simulink model "Furuta_Pendulum_Classical_Controller"  (R2018a)
settings: Solver=VariableStepAuto  StartTime=0.0  StopTime=10.0  RelTol=1e-3
values from neighbouring files (symbols this model uses):
  Ac = [0 1 0 0 ... (first row only)    [BasicModelParameters.m]    (also in ControllerDesign_REV0.m; FurutaPendulum.m = [0 1 0 0; 0 0 -a23 0; 0 0 0 1; 0 0 a43 0]; InvertedPendulumStepResponse.m)
  Bc = transpose([0 b21 0 -b41])    [BasicModelParameters.m]    (also in ControllerDesign_REV0.m; FurutaPendulum.m = [0; b21; 0; -b41]; InvertedPendulumStepResponse.m)
  Cc = [1 0 0 0 ... (first row only)    [BasicModelParameters.m]    (also in ControllerDesign_REV0.m; FurutaPendulum.m = [1 0 0 0; 0 0 1 0]; InvertedPendulumStepResponse.m)
  Dc = [0 ... (first row only)    [BasicModelParameters.m]    (also in ControllerDesign_REV0.m; FurutaPendulum.m = [0; 0]; InvertedPendulumStepResponse.m)
settings Model: Creator=jcarroll  LastModifiedBy=Jack

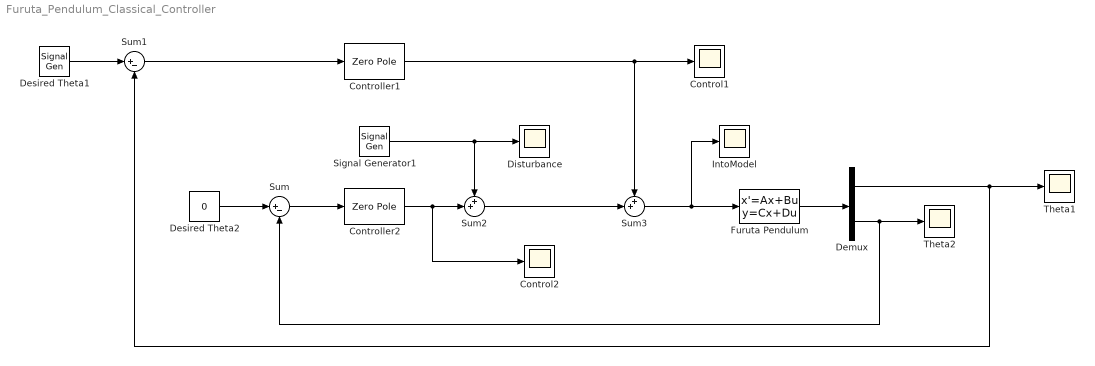
== system Furuta_Pendulum_Classical_Controller ==
  Control1 : Scope
  Control2 : Scope
  Controller1 : ZeroPole  Zeros=[-0.1229, -0.02181]  Poles=[-284.8, 0]  Gain=[-5.2947]
  Controller2 : ZeroPole  Zeros=[-9.249]  Poles=[-50]  Gain=[-5.1415]
  Demux : Demux  Outputs=2
  Desired Theta1 : SignalGenerator  Amplitude=pi/4  Frequency=.1
  Desired Theta2 : Constant  Value=0
  Disturbance : Scope
  Furuta Pendulum : StateSpace  A=Ac  B=Bc  C=Cc  D=Dc  InitialCondition=[0; 0; 0.05; 0]  ContinuousStateAttributes='Theta'
  IntoModel : Scope
  Signal Generator1 : SignalGenerator  WaveForm=square  Amplitude=0
  Sum : Sum  Inputs=|+-
  Sum1 : Sum  Inputs=|+-
  Sum2 : Sum  Inputs=++|
  Sum3 : Sum  Inputs=++|
  Theta1 : Scope
  "Theta2 " : Scope
  wires:
  Furuta Pendulum/1 -> Demux/1
  Sum/1 -> Controller2/1
  Demux/2 -> Sum/2, "Theta2 "/1
  Desired Theta2/1 -> Sum/1
  Controller2/1 -> Control2/1, Sum2/2
  Demux/1 -> Sum1/2, Theta1/1
  Desired Theta1/1 -> Sum1/1
  Signal Generator1/1 -> Disturbance/1, Sum2/1
  Sum2/1 -> Sum3/2
  Sum3/1 -> IntoModel/1, Furuta Pendulum/1
  Sum1/1 -> Controller1/1
  Controller1/1 -> Control1/1, Sum3/1
